simulink model "RLC"  (R2020b)
settings: Solver=VariableStepAuto  StartTime=0.0  StopTime=Endtime  RelTol=1e-3
values from neighbouring files (symbols this model uses):
  C = 100e-6    (= 0.0001)    [RLC_sim.m]
  L = 100e-3    (= 0.1)    [RLC_sim.m]
  R = 100    [RLC_sim.m]
  v = 5    [RLC_sim.m]
settings Model: Creator=yuto  LastModifiedBy=yuto

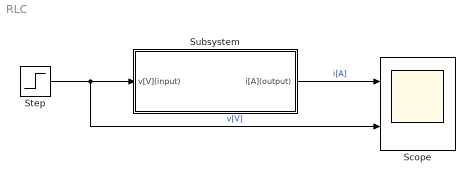
== system RLC ==
  Scope : Scope  NumInputPorts=2
  Step : Step  Time=0.1  After=v  SampleTime=0
  Subsystem : Subsystem
  wires:
  Step/1 -> Scope/2, Subsystem/1(v[V](input))  "v[V]"
  Subsystem/1(i[A](output)) -> Scope/1  "i[A]"

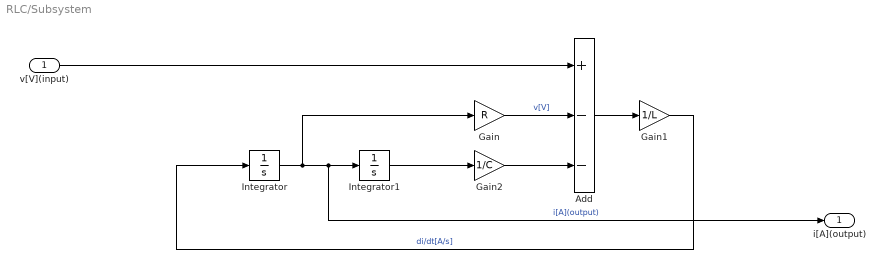
== system RLC/Subsystem ==
  v[V](input) : Inport
  Add : Sum  Inputs=+--
  Gain : Gain  Gain=R
  Gain1 : Gain  Gain=1/L
  Gain2 : Gain  Gain=1/C
  Integrator : Integrator
  Integrator1 : Integrator
  i[A](output) : Outport
  wires:
  Gain2/1 -> Add/3
  Integrator/1 -> Gain/1, i[A](output)/1, Integrator1/1  "i[A](output)"
  Add/1 -> Gain1/1
  Integrator1/1 -> Gain2/1
  v[V](input)/1 -> Add/1
  Gain1/1 -> Integrator/1  "di/dt[A/s]"
  Gain/1 -> Add/2  "v[V]"
